simulink library "BatteryPack_lib"  (R2022b)
settings: Solver=VariableStepAuto  StartTime=0.0  StopTime=10.0  RelTol=1e-3
undefined symbols (not defined in the file or in its folder): Battery, ts
libraries: fl_lib x78, nesl_utility x48, simulink x16, batteryecm_lib x14, ee_lib x4
(part 2 of 2)

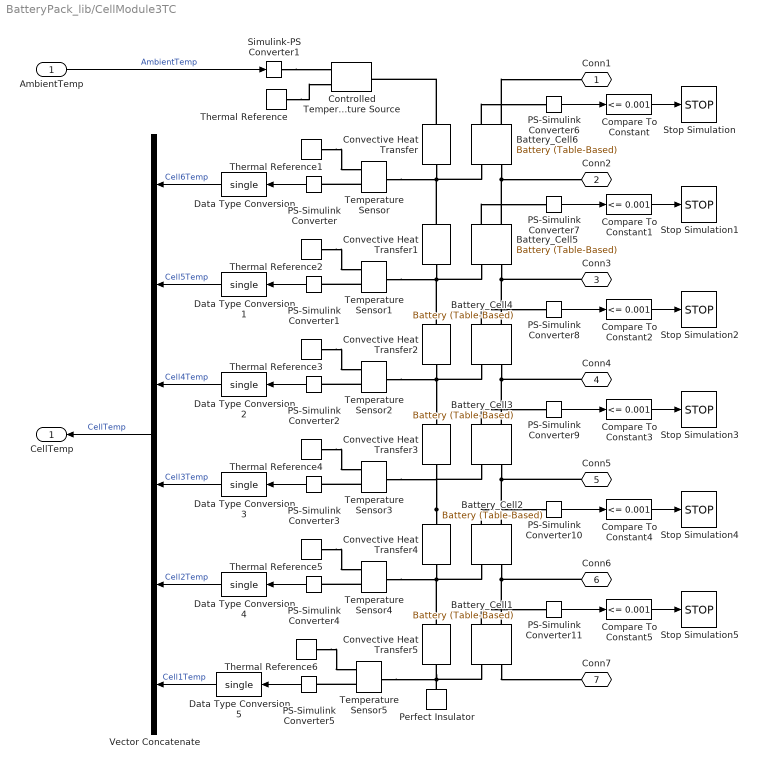
== system BatteryPack_lib/CellModule3TC ==
  AmbientTemp : Inport
  Battery_Cell{1..6} (6 alike) : batteryecm_lib/Battery (Table-Based)  SOC_vec=Battery.SOC_LUT  T_dependence=simscape.enum.tablebattery.temperature_dependence.yes  prm_dir=simscape.enum.tablebattery.prm_dir.noCurrentDirectionality  T_vec=Battery.Temperature_LUT K  V0_mat=Battery.Em_LUT V  V0_vec=[3.1, 3.27, 3.31, 3.5] V  V_range=[0, inf] V  R0_mat=Battery.R0_LUT Ohm  R0_vec=[.015, .017, .012, .013] Ohm  R0_dis_mat=[.0117, .0085, .009; .011, .0085, .009; .0114, .0087, .0092; .0107, .0082, .0088; .0107, .0083, .0091; .0113, .0085, .0089; .0116, .0085, .0089] Ohm  R0_dis_vec=[.0085, .0085, .0087, .0082, .0083, .0085, .0085] Ohm  R0_ch_mat=[.0117, .0085, .009; .011, .0085, .009; .0114, .0087, .0092; .0107, .0082, .0088; .0107, .0083, .0091; .0113, .0085, .0089; .0116, .0085, .0089] Ohm  R0_ch_vec=[.0085, .0085, .0087, .0082, .0083, .0085, .0085] Ohm  AH=Battery.Capacity_LUT hr*A  prm_leak=1  Rleak_vec=[8000, 7000, 6000] Ohm  Rleak=7e3 Ohm  extrapolation_option=simscape.enum.extrapolation.linear  SOC_port=simscape.enum.tablebattery.enable.yes  prm_dyn=4  R1_mat=Battery.R1_LUT Ohm  R1_vec=[.076, .022, .007, .043] Ohm  tau1_mat=Battery.R1_LUT.*Battery.C1_LUT s  tau1_vec=[148, 110, 27, 22] s  R2_mat=Battery.R2_LUT Ohm  R2_vec=[.382, .006, .007, .956] Ohm  tau2_mat=Battery.R2_LUT.*Battery.C2_LUT s  tau2_vec=[44, 24, 14, 13419] s  R3_mat=Battery.R3_LUT Ohm  R3_vec=[.382, .006, .007, .956] Ohm  tau3_mat=Battery.R3_LUT.*Battery.C3_LUT s  tau3_vec=[44, 24, 14, 13419] s  R4_mat=[.014, .382, .407; .028, .006, .007; .014, .007, .006; .333, .956, .912] Ohm  R4_vec=[.382, .006, .007, .956] Ohm  tau4_mat=[1, 44, 5644; 11, 24, 506; 2, 14, 330; 3310, 13419, 30216] s  tau4_vec=[44, 24, 14, 13419] s  R5_mat=[.014, .382, .407; .028, .006, .007; .014, .007, .006; .333, .956, .912] Ohm  R5_vec=[.382, .006, .007, .956] Ohm  tau5_mat=[1, 44, 5644; 11, 24, 506; 2, 14, 330; 3310, 13419, 30216] s  tau5_vec=[44, 24, 14, 13419] s  prm_fade=simscape.enum.tablebattery.prm_fade.equations  N0=100  dV0=0  dR0=0  dAH=0  dRleak=0  dR1=0  dR2=0  dR3=0  dR4=0  dR5=0  N0vec=[100, 200, 300]  Tfadevec=[298.15, 323.15] K  dV0vec=[0, 0, 0]  dR0vec=[0, 0, 0]  dAHvec=[0, 0, 0]  dRleakvec=[0, 0, 0]  dR1vec=[0, 0, 0]  dR2vec=[0, 0, 0]  dR3vec=[0, 0, 0]  dR4vec=[0, 0, 0]  dR5vec=[0, 0, 0]  dV0mat=[0, 0; 0, 0; 0, 0]  dR0mat=[0, 0; 0, 0; 0, 0]  dAHmat=[0, 0; 0, 0; 0, 0]  dRleakmat=[0, 0; 0, 0; 0, 0]  dR1mat=[0, 0; 0, 0; 0, 0]  dR2mat=[0, 0; 0, 0; 0, 0]  dR3mat=[0, 0; 0, 0; 0, 0]  dR4mat=[0, 0; 0, 0; 0, 0]  dR5mat=[0, 0; 0, 0; 0, 0]  prm_age_modeling=simscape.enum.tablebattery.prm_age_modeling.equation  storage_dt_age_vec=[0] d  storage_T_age_vec=[273] K  prm_age_OCV=simscape.enum.tablebattery.prm_age_OCV.OCV  OCV_age=0.9  SOC_age=0.6  prm_age_resistance=simscape.enum.tablebattery.prm_age.disabled  OCV_scaling_age_resistance=2.2134e6  OCV_offset_age_resistance=1.632e6  temp_exp_age_resistance=0.515833569 V  t_exp_age_resistance=0.75  T_age_vec_resistance=[273.15, 298.15, 323.15] K  dt_age_vec_resistance=[90, 180, 270, 360] d  dR0_age_vec=[0, 0, 0]  t_meas_dR0_age=100 d  dR0_age_mat=[0, 0, 0; 0, 0, 0; 0, 0, 0; 0, 0, 0]  prm_age_capacity=simscape.enum.tablebattery.prm_age.disabled  OCV_scaling_age_capacity=1.5097e07  OCV_offset_age_capacity=8.3625e06  temp_exp_age_capacity=0.6011 V  t_exp_age_capacity=0.75  T_age_vec_capacity=[273.15, 298.15, 323.15] K  dt_age_vec_capacity=[90, 180, 270, 360] d  dAH_age_vec=[0, 0, 0]  t_meas_dAH_age=100 d  dAH_age_mat=[0, 0, 0; 0, 0, 0; 0, 0, 0; 0, 0, 0]  thermal_port=simscape.enum.thermaleffects.model  temperature=Battery.TempInit K  thermal_mass=Battery.cell_mass*Battery.cell_Cp_heat J/K  i_specify=off  i_priority=None  i=0 A  i_nominal_specify=off  i_nominal_unit=A  i_nominal_value=1  v_specify=off  v_priority=None  v=0 V  v_nominal_specify=off  v_nominal_unit=V  v_nominal_value=1  stateOfCharge_specify=on  stateOfCharge_priority=High  stateOfCharge=(Battery.Capacity_LUT - Battery.Qe_init)/Battery.Capacity_LUT  stateOfCharge_nominal_specify=off  stateOfCharge_nominal_unit=1  stateOfCharge_nominal_value=1  num_cycles_specify=off  num_cycles_priority=High  num_cycles=0  num_cycles_nominal_specify=off  num_cycles_nominal_unit=1  num_cycles_nominal_value=1  cell_temperature_specify=on  cell_temperature_priority=High  cell_temperature=Battery.TempInit K  cell_temperature_nominal_specify=off  cell_temperature_nominal_unit=K  cell_temperature_nominal_value=1
  Compare To Constant{,1..5} (6 alike) : simulink/Logic and Bit Operations/Compare To Constant  relop=<=  const=0.001  OutDataTypeStr=boolean
  Controlled Temperature Source : fl_lib/Thermal/Thermal Sources/Controlled Temperature Source
  Convective Heat Transfer{,1..5} (6 alike) : fl_lib/Thermal/Thermal Elements/Convective Heat Transfer  thermal_type=foundation.enum.constant_variable.constant  area=Battery.cell_area m^2  heat_tr_coeff=Battery.h_conv W/(m^2 * K)  min_heat_tr_coeff=1e-3 W/(K*m^2)  T_specify=off  T_priority=None  T=0 K  T_nominal_specify=off  T_nominal_unit=K  T_nominal_value=1  Q_specify=off  Q_priority=None  Q=0 W  Q_nominal_specify=off  Q_nominal_unit=W  Q_nominal_value=1
  Data Type Conversion{,1..5} (6 alike) : DataTypeConversion  OutDataTypeStr=single  SaturateOnIntegerOverflow=off  RndMeth=Floor
  PS-Simulink Converter{,1..5} (6 alike) : nesl_utility/PS-Simulink Converter  PhysicalDomain=network_engine_domain  SubClassName=ps_output  LeftPortType=input  RightPortType=output  PseudoPeriodic=off  Frequencies=[]  VectorFormat=1-D array  Unit=K  AffineConversion=off
  PS-Simulink Converter{6..11} (6 alike) : nesl_utility/PS-Simulink Converter  PhysicalDomain=network_engine_domain  SubClassName=ps_output  LeftPortType=input  RightPortType=output  PseudoPeriodic=off  Frequencies=[]  VectorFormat=1-D array  Unit=1  AffineConversion=off
  Perfect Insulator : fl_lib/Thermal/Thermal Elements/Perfect Insulator  T_specify=off  T_priority=None  T=0 K  T_nominal_specify=off  T_nominal_unit=K  T_nominal_value=1
  Simulink-PS Converter1 : nesl_utility/Simulink-PS Converter  PhysicalDomain=network_engine_domain  SubClassName=ps_input  LeftPortType=input  RightPortType=output  PseudoPeriodic=off  Frequencies=[]  NoiseDistribution=none  NoiseParameters=[]  Unit=1  AffineConversion=off  FilteringAndDerivatives=provide  SimscapeFilterOrder=1  InputFilterTimeConstant=0.001  UdotUserProvided=0
  Stop Simulation{,1..5} (6 alike) : Stop
  Temperature Sensor{,1..5} (6 alike) : fl_lib/Thermal/Thermal Sensors/Temperature Sensor
  Thermal Reference{,1..6} (7 alike) : fl_lib/Thermal/Thermal Elements/Thermal Reference
  Vector Concatenate : Concatenate  NumInputs=6
  Conn1 : PMIOPort  Side=Right
  Conn2 : PMIOPort  Port=2  Side=Right
  Conn3 : PMIOPort  Port=3  Side=Right
  Conn4 : PMIOPort  Port=4  Side=Right
  Conn5 : PMIOPort  Port=5  Side=Right
  Conn6 : PMIOPort  Port=6  Side=Right
  Conn7 : PMIOPort  Port=7  Side=Right
  CellTemp : Outport  VectorParamsAs1DForOutWhenUnconnected=off
  wires:
  Compare To Constant3/1 -> Stop Simulation3/1
  Data Type Conversion4/1 -> Vector Concatenate/5  "Cell2Temp"
  Compare To Constant5/1 -> Stop Simulation5/1
  Data Type Conversion5/1 -> Vector Concatenate/6  "Cell1Temp"
  PS-Simulink Converter2/1 -> Data Type Conversion2/1
  Compare To Constant1/1 -> Stop Simulation1/1
  PS-Simulink Converter11/1 -> Compare To Constant5/1
  Data Type Conversion1/1 -> Vector Concatenate/2  "Cell5Temp"
  Compare To Constant4/1 -> Stop Simulation4/1
  Data Type Conversion2/1 -> Vector Concatenate/3  "Cell4Temp"
  Data Type Conversion3/1 -> Vector Concatenate/4  "Cell3Temp"
  PS-Simulink Converter8/1 -> Compare To Constant2/1
  PS-Simulink Converter3/1 -> Data Type Conversion3/1
  PS-Simulink Converter1/1 -> Data Type Conversion1/1
  PS-Simulink Converter9/1 -> Compare To Constant3/1
  PS-Simulink Converter4/1 -> Data Type Conversion4/1
  PS-Simulink Converter10/1 -> Compare To Constant4/1
  PS-Simulink Converter7/1 -> Compare To Constant1/1
  PS-Simulink Converter5/1 -> Data Type Conversion5/1
  Compare To Constant/1 -> Stop Simulation/1
  PS-Simulink Converter/1 -> Data Type Conversion/1
  Data Type Conversion/1 -> Vector Concatenate/1  "Cell6Temp"
  Compare To Constant2/1 -> Stop Simulation2/1
  AmbientTemp/1 -> Simulink-PS Converter1/1  "AmbientTemp"
  Vector Concatenate/1 -> CellTemp/1  "CellTemp"
  PS-Simulink Converter6/1 -> Compare To Constant/1
  connections:
  Battery_Cell3/RConn1 -- Conn5/RConn1 -- Battery_Cell2/LConn1
  Temperature Sensor2/RConn2 -- PS-Simulink Converter2/LConn1
  Battery_Cell1/LConn2 -- PS-Simulink Converter11/LConn1
  Temperature Sensor1/RConn2 -- PS-Simulink Converter1/LConn1
  Battery_Cell2/RConn1 -- Conn6/RConn1 -- Battery_Cell1/LConn1
  Battery_Cell4/RConn1 -- Conn4/RConn1 -- Battery_Cell3/LConn1
  Convective Heat Transfer/LConn1 -- Controlled Temperature Source/LConn1
  Thermal Reference1/LConn1 -- Temperature Sensor/RConn1
  Convective Heat Transfer1/LConn1 -- Temperature Sensor/LConn1 -- Convective Heat Transfer/RConn1 -- Battery_Cell6/RConn2
  Convective Heat Transfer5/LConn1 -- Temperature Sensor4/LConn1 -- Convective Heat Transfer4/RConn1 -- Battery_Cell2/RConn2
  Battery_Cell6/RConn1 -- Conn2/RConn1 -- Battery_Cell5/LConn1
  Perfect Insulator/LConn1 -- Temperature Sensor5/LConn1 -- Convective Heat Transfer5/RConn1 -- Battery_Cell1/RConn2
  Thermal Reference3/LConn1 -- Temperature Sensor2/RConn1
  Temperature Sensor/RConn2 -- PS-Simulink Converter/LConn1
  Convective Heat Transfer4/LConn1 -- Temperature Sensor3/LConn1 -- Convective Heat Transfer3/RConn1 -- Battery_Cell3/RConn2
  Battery_Cell1/RConn1 -- Conn7/RConn1
  Battery_Cell6/LConn1 -- Conn1/RConn1
  Battery_Cell6/LConn2 -- PS-Simulink Converter6/LConn1
  Thermal Reference4/LConn1 -- Temperature Sensor3/RConn1
  Temperature Sensor3/RConn2 -- PS-Simulink Converter3/LConn1
  Thermal Reference5/LConn1 -- Temperature Sensor4/RConn1
  Thermal Reference/LConn1 -- Controlled Temperature Source/RConn2
  Temperature Sensor4/RConn2 -- PS-Simulink Converter4/LConn1
  Battery_Cell4/RConn2 -- Temperature Sensor2/LConn1 -- Convective Heat Transfer2/RConn1 -- Convective Heat Transfer3/LConn1
  Temperature Sensor5/RConn2 -- PS-Simulink Converter5/LConn1
  Thermal Reference6/LConn1 -- Temperature Sensor5/RConn1
  Battery_Cell5/RConn1 -- Conn3/RConn1 -- Battery_Cell4/LConn1
  Battery_Cell5/LConn2 -- PS-Simulink Converter7/LConn1
  Convective Heat Transfer2/LConn1 -- Temperature Sensor1/LConn1 -- Convective Heat Transfer1/RConn1 -- Battery_Cell5/RConn2
  Battery_Cell3/LConn2 -- PS-Simulink Converter9/LConn1
  Battery_Cell4/LConn2 -- PS-Simulink Converter8/LConn1
  Battery_Cell2/LConn2 -- PS-Simulink Converter10/LConn1
  Thermal Reference2/LConn1 -- Temperature Sensor1/RConn1
  Simulink-PS Converter1/RConn1 -- Controlled Temperature Source/RConn1

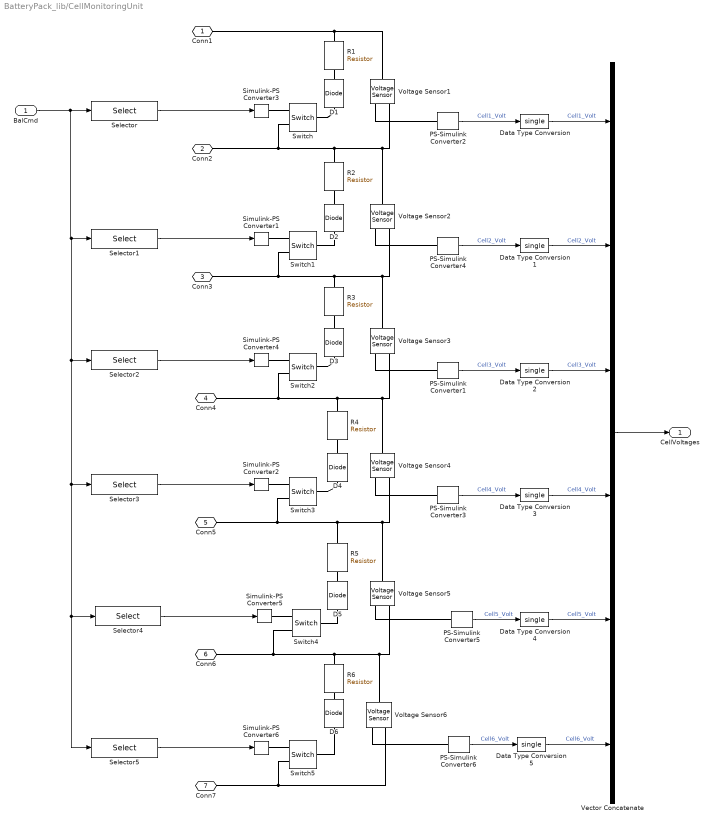
== system BatteryPack_lib/CellMonitoringUnit ==
  BalCmd : Inport
  D{1..4} (4 alike) : fl_lib/Electrical/Electrical Elements/Diode  Vf=0.6 V  Ron=0.3 Ohm  Goff=1e-8 1/Ohm  i_specify=off  i_priority=High  i=0 A  i_nominal_specify=off  i_nominal_unit=A  i_nominal_value=1  v_specify=off  v_priority=None  v=0 V  v_nominal_specify=off  v_nominal_unit=V  v_nominal_value=1
      settings: LogSimulationData=on
  D5 : fl_lib/Electrical/Electrical Elements/Diode  Vf=0.6 V  Ron=0.3 Ohm  Goff=1e-8 1/Ohm  i_specify=off  i_priority=None  i=0 A  i_nominal_specify=off  i_nominal_unit=A  i_nominal_value=1  v_specify=off  v_priority=None  v=0 V  v_nominal_specify=off  v_nominal_unit=V  v_nominal_value=1
      settings: LogSimulationData=on
  D6 : fl_lib/Electrical/Electrical Elements/Diode  Vf=0.6 V  Ron=0.3 Ohm  Goff=1e-8 1/Ohm  i_specify=off  i_priority=None  i=0 A  i_nominal_specify=off  i_nominal_unit=A  i_nominal_value=1  v_specify=off  v_priority=None  v=0 V  v_nominal_specify=off  v_nominal_unit=V  v_nominal_value=1
      settings: LogSimulationData=on
  Data Type Conversion{,1..5} (6 alike) : DataTypeConversion  OutDataTypeStr=single  SaturateOnIntegerOverflow=off  RndMeth=Floor
  PS-Simulink Converter{1..6} (6 alike) : nesl_utility/PS-Simulink Converter  PhysicalDomain=network_engine_domain  SubClassName=ps_output  LeftPortType=input  RightPortType=output  PseudoPeriodic=off  Frequencies=[]  VectorFormat=1-D array  Unit=V  AffineConversion=off
  R{1..6} (6 alike) : fl_lib/Electrical/Electrical Elements/Resistor  R=Battery.R_bleed Ohm  i_specify=off  i_priority=None  i=0 A  i_nominal_specify=off  i_nominal_unit=A  i_nominal_value=1  v_specify=off  v_priority=None  v=0 V  v_nominal_specify=off  v_nominal_unit=V  v_nominal_value=1
      R1 settings: LogSimulationData=on
  Selector : Selector  IndexOptions=Index vector (dialog)  Indices=1  OutputSizes=1
  Selector1 : Selector  IndexOptions=Index vector (dialog)  Indices=2  OutputSizes=1
  Selector2 : Selector  IndexOptions=Index vector (dialog)  Indices=3  OutputSizes=1
  Selector3 : Selector  IndexOptions=Index vector (dialog)  Indices=4  OutputSizes=1
  Selector4 : Selector  IndexOptions=Index vector (dialog)  Indices=5  OutputSizes=1
  Selector5 : Selector  IndexOptions=Index vector (dialog)  Indices=6  OutputSizes=1
  Simulink-PS Converter{1..6} (6 alike) : nesl_utility/Simulink-PS Converter  PhysicalDomain=network_engine_domain  SubClassName=ps_input  LeftPortType=input  RightPortType=output  PseudoPeriodic=off  Frequencies=[]  NoiseDistribution=none  NoiseParameters=[]  Unit=1  AffineConversion=off  FilteringAndDerivatives=zero  SimscapeFilterOrder=1  InputFilterTimeConstant=0.001  UdotUserProvided=1
  Switch{,1..5} (6 alike) : fl_lib/Electrical/Electrical Elements/Switch  R_closed=0.01 Ohm  G_open=1e-8 1/Ohm  Threshold=0  i_specify=off  i_priority=None  i=0 A  i_nominal_specify=off  i_nominal_unit=A  i_nominal_value=1  v_specify=off  v_priority=None  v=0 V  v_nominal_specify=off  v_nominal_unit=V  v_nominal_value=1
  Vector Concatenate : Concatenate  NumInputs=6
  Voltage Sensor{1..6} (6 alike) : fl_lib/Electrical/Electrical Sensors/Voltage Sensor
  Conn1 : PMIOPort  Side=Left
  Conn2 : PMIOPort  Port=2  Side=Left
  Conn3 : PMIOPort  Port=3  Side=Left
  Conn4 : PMIOPort  Port=4  Side=Left
  Conn5 : PMIOPort  Port=5  Side=Left
  Conn6 : PMIOPort  Port=6  Side=Left
  Conn7 : PMIOPort  Port=7  Side=Left
  CellVoltages : Outport  VectorParamsAs1DForOutWhenUnconnected=off
  wires:
  Vector Concatenate/1 -> CellVoltages/1
  Selector2/1 -> Simulink-PS Converter4/1
  Selector1/1 -> Simulink-PS Converter1/1
  BalCmd/1 -> Selector5/1, Selector4/1, Selector3/1, Selector2/1, Selector1/1, Selector/1
  PS-Simulink Converter2/1 -> Data Type Conversion/1  "Cell1_Volt"
  PS-Simulink Converter1/1 -> Data Type Conversion2/1  "Cell3_Volt"
  PS-Simulink Converter4/1 -> Data Type Conversion1/1  "Cell2_Volt"
  Selector/1 -> Simulink-PS Converter3/1
  Selector3/1 -> Simulink-PS Converter2/1
  Selector4/1 -> Simulink-PS Converter5/1
  Selector5/1 -> Simulink-PS Converter6/1
  PS-Simulink Converter3/1 -> Data Type Conversion3/1  "Cell4_Volt"
  PS-Simulink Converter5/1 -> Data Type Conversion4/1  "Cell5_Volt"
  PS-Simulink Converter6/1 -> Data Type Conversion5/1  "Cell6_Volt"
  Data Type Conversion/1 -> Vector Concatenate/1  "Cell1_Volt"
  Data Type Conversion1/1 -> Vector Concatenate/2  "Cell2_Volt"
  Data Type Conversion2/1 -> Vector Concatenate/3  "Cell3_Volt"
  Data Type Conversion3/1 -> Vector Concatenate/4  "Cell4_Volt"
  Data Type Conversion4/1 -> Vector Concatenate/5  "Cell5_Volt"
  Data Type Conversion5/1 -> Vector Concatenate/6  "Cell6_Volt"
  connections:
  Voltage Sensor3/RConn2 -- Voltage Sensor4/LConn1 -- R4/LConn1 -- Conn4/RConn1 -- Switch2/RConn2
  Voltage Sensor3/RConn1 -- PS-Simulink Converter1/LConn1
  Simulink-PS Converter4/RConn1 -- Switch2/RConn1
  Simulink-PS Converter1/RConn1 -- Switch1/RConn1
  Simulink-PS Converter3/RConn1 -- Switch/RConn1
  Switch1/LConn1 -- D2/RConn1
  Voltage Sensor2/RConn1 -- PS-Simulink Converter4/LConn1
  PS-Simulink Converter2/LConn1 -- Voltage Sensor1/RConn1
  Conn1/RConn1 -- Voltage Sensor1/LConn1 -- R1/LConn1
  Switch2/LConn1 -- D3/RConn1
  Switch/LConn1 -- D1/RConn1
  R2/RConn1 -- D2/LConn1
  R1/RConn1 -- D1/LConn1
  Conn2/RConn1 -- Voltage Sensor1/RConn2 -- Voltage Sensor2/LConn1 -- R2/LConn1 -- Switch/RConn2
  Voltage Sensor2/RConn2 -- Voltage Sensor3/LConn1 -- Conn3/RConn1 -- Switch1/RConn2 -- R3/LConn1
  R3/RConn1 -- D3/LConn1
  R5/LConn1 -- Conn5/RConn1 -- Switch3/RConn2 -- Voltage Sensor5/LConn1 -- Voltage Sensor4/RConn2
  R4/RConn1 -- D4/LConn1
  Switch3/LConn1 -- D4/RConn1
  Simulink-PS Converter2/RConn1 -- Switch3/RConn1
  Conn6/RConn1 -- Switch4/RConn2 -- Voltage Sensor5/RConn2 -- Voltage Sensor6/LConn1 -- R6/LConn1
  Simulink-PS Converter5/RConn1 -- Switch4/RConn1
  R5/RConn1 -- D5/LConn1
  Switch4/LConn1 -- D5/RConn1
  Voltage Sensor6/RConn2 -- Conn7/RConn1 -- Switch5/RConn2
  Switch5/LConn1 -- D6/RConn1
  Simulink-PS Converter6/RConn1 -- Switch5/RConn1
  R6/RConn1 -- D6/LConn1
  Voltage Sensor4/RConn1 -- PS-Simulink Converter3/LConn1
  Voltage Sensor5/RConn1 -- PS-Simulink Converter5/LConn1
  Voltage Sensor6/RConn1 -- PS-Simulink Converter6/LConn1

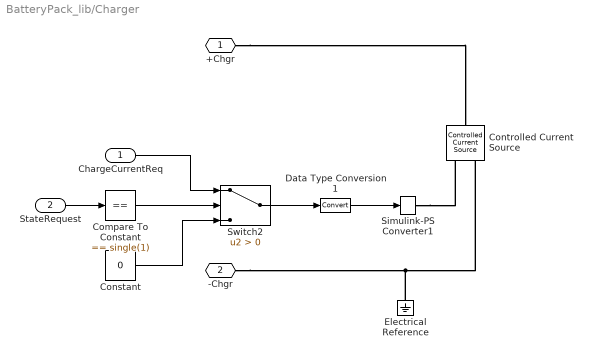
== system BatteryPack_lib/Charger ==
  ChargeCurrentReq : Inport
  StateRequest : Inport  Port=2
  Compare To Constant : simulink/Logic and Bit Operations/Compare To Constant  relop===  const=single(1)  OutDataTypeStr=boolean
  Constant : Constant  Value=0  SampleTime=ts
  Controlled Current Source : fl_lib/Electrical/Electrical Sources/Controlled Current Source
      settings: LogSimulationData=on
  Data Type Conversion1 : DataTypeConversion  SaturateOnIntegerOverflow=off  RndMeth=Floor
  Electrical Reference : fl_lib/Electrical/Electrical Elements/Electrical Reference
  Simulink-PS Converter1 : nesl_utility/Simulink-PS Converter  PhysicalDomain=network_engine_domain  SubClassName=ps_input  LeftPortType=input  RightPortType=output  PseudoPeriodic=off  Frequencies=[]  NoiseDistribution=none  NoiseParameters=[]  Unit=A  AffineConversion=off  FilteringAndDerivatives=zero  SimscapeFilterOrder=1  InputFilterTimeConstant=0.1  UdotUserProvided=1
  Switch2 : Switch  Criteria=u2 > Threshold  SaturateOnIntegerOverflow=off  InputSameDT=off
  +Chgr : PMIOPort  Side=Left
  -Chgr : PMIOPort  Port=2  Side=Left
  wires:
  Compare To Constant/1 -> Switch2/2
  Switch2/1 -> Data Type Conversion1/1
  Constant/1 -> Switch2/3
  StateRequest/1 -> Compare To Constant/1
  Data Type Conversion1/1 -> Simulink-PS Converter1/1
  ChargeCurrentReq/1 -> Switch2/1
  connections:
  +Chgr/RConn1 -- Controlled Current Source/LConn1
  Controlled Current Source/RConn2 -- -Chgr/RConn1 -- Electrical Reference/LConn1
  Simulink-PS Converter1/RConn1 -- Controlled Current Source/RConn1

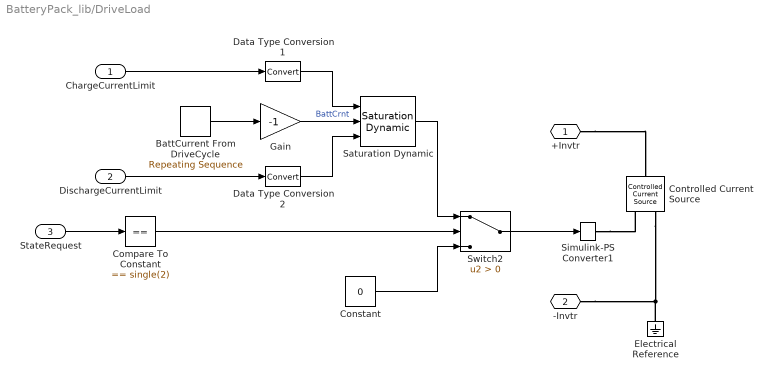
== system BatteryPack_lib/DriveLoad ==
  ChargeCurrentLimit : Inport
  DischargeCurrentLimit : Inport  Port=2
  StateRequest : Inport  Port=3
  BattCurrent From DriveCycle : simulink/Sources/Repeating Sequence  rep_seq_t=BattCrnt.Time  rep_seq_y=BattCrnt.Data
  Compare To Constant : simulink/Logic and Bit Operations/Compare To Constant  relop===  const=single(2)  OutDataTypeStr=boolean
  Constant : Constant  Value=0  SampleTime=ts
  Controlled Current Source : fl_lib/Electrical/Electrical Sources/Controlled Current Source
      settings: LogSimulationData=on
  Data Type Conversion1 : DataTypeConversion  SaturateOnIntegerOverflow=off  RndMeth=Floor
  Data Type Conversion2 : DataTypeConversion  SaturateOnIntegerOverflow=off  RndMeth=Floor
  Electrical Reference : fl_lib/Electrical/Electrical Elements/Electrical Reference
  Gain : Gain  Gain=-1
  Saturation Dynamic : simulink/Discontinuities/Saturation Dynamic  OutMin=[]  OutMax=[]  OutDataTypeStr=Inherit: Same as second input  OutDataType=fixdt(1, 16)  OutScaling=2^-10  DoSatur=off
  Simulink-PS Converter1 : nesl_utility/Simulink-PS Converter  PhysicalDomain=network_engine_domain  SubClassName=ps_input  LeftPortType=input  RightPortType=output  PseudoPeriodic=off  Frequencies=[]  NoiseDistribution=none  NoiseParameters=[]  Unit=A  AffineConversion=off  FilteringAndDerivatives=zero  SimscapeFilterOrder=1  InputFilterTimeConstant=0.1  UdotUserProvided=1
  Switch2 : Switch  Criteria=u2 > Threshold  SaturateOnIntegerOverflow=off  InputSameDT=off
  +Invtr : PMIOPort  Side=Left
  -Invtr : PMIOPort  Port=2  Side=Left
  wires:
  BattCurrent From DriveCycle/1 -> Gain/1
  Gain/1 -> Saturation Dynamic/2  "BattCrnt"
  Compare To Constant/1 -> Switch2/2
  StateRequest/1 -> Compare To Constant/1
  Switch2/1 -> Simulink-PS Converter1/1
  Constant/1 -> Switch2/3
  Data Type Conversion2/1 -> Saturation Dynamic/3
  Data Type Conversion1/1 -> Saturation Dynamic/1
  ChargeCurrentLimit/1 -> Data Type Conversion1/1
  DischargeCurrentLimit/1 -> Data Type Conversion2/1
  Saturation Dynamic/1 -> Switch2/1
  connections:
  Simulink-PS Converter1/RConn1 -- Controlled Current Source/RConn1
  -Invtr/RConn1 -- Electrical Reference/LConn1 -- Controlled Current Source/RConn2
  +Invtr/RConn1 -- Controlled Current Source/LConn1

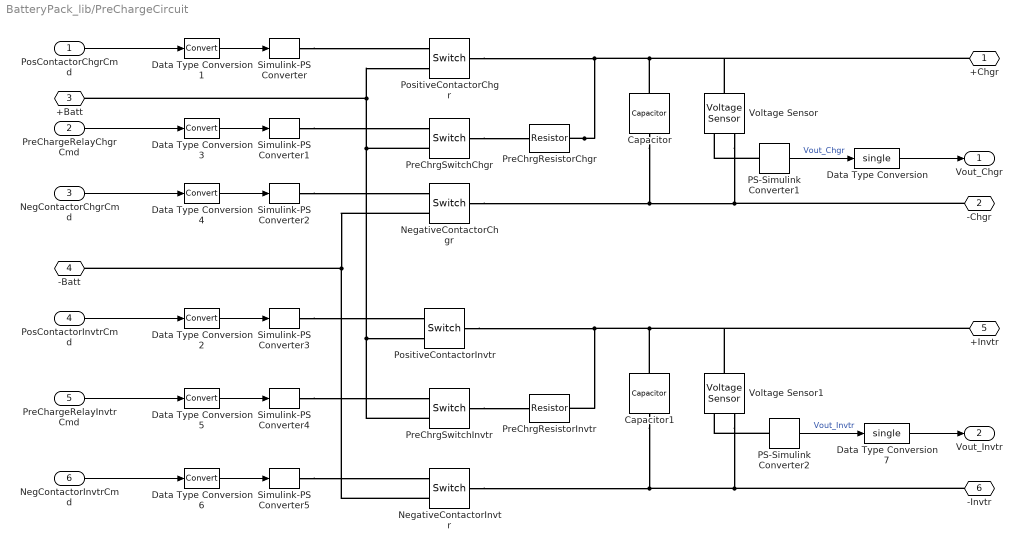
== system BatteryPack_lib/PreChargeCircuit ==
  PosContactorChgrCmd : Inport
  PreChargeRelayChgrCmd : Inport  Port=2
  NegContactorChgrCmd : Inport  Port=3
  PosContactorInvtrCmd : Inport  Port=4
  PreChargeRelayInvtrCmd : Inport  Port=5
  NegContactorInvtrCmd : Inport  Port=6
  Capacitor : ee_lib/Passive/Capacitor  cap_option=0  c=10000 uF  Cvec=[1e-05, 1e-06] F  Vvec=[0, 10] V  CV_table_symmetry=1  f_vec=[1, 10] kHz  DFext_vec=[.8, 1.2]  enable_C_tol=0  C_tol=5  tol_distribution=1  nSigma=4  r=1e-9 Ohm  g=0 1/Ohm  averaging_period=0 s  enable_operating_limits=0  operating_limit_action=2  max_working_voltage_range=[-25, 25] V  power_rating=1 W  enable_faults=0  fault_action=1  Cscale_faulted=100  R_faulted=1e-3 Ohm  G_faulted=0 1/Ohm  tau_fault=1e-3 s  enable_temporal_fault=0  t_fault=1 s  enable_behavioral_fault=0  max_permissible_voltage_range=[-100, 100] V  t_fail_on_voltage=1 s  i_specify=off  i_priority=None  i=0 A  i_nominal_specify=off  i_nominal_unit=A  i_nominal_value=1  v_specify=off  v_priority=None  v=0 V  v_nominal_specify=off  v_nominal_unit=V  v_nominal_value=1  vc_specify=off  vc_priority=High  vc=0 V  vc_nominal_specify=off  vc_nominal_unit=V  vc_nominal_value=1
  Capacitor1 : ee_lib/Passive/Capacitor  cap_option=0  c=10000 uF  Cvec=[1e-05, 1e-06] F  Vvec=[0, 10] V  CV_table_symmetry=1  f_vec=[1, 10] kHz  DFext_vec=[.8, 1.2]  enable_C_tol=0  C_tol=5  tol_distribution=1  nSigma=4  r=1e-9 Ohm  g=0 1/Ohm  averaging_period=0 s  enable_operating_limits=0  operating_limit_action=2  max_working_voltage_range=[-25, 25] V  power_rating=1 W  enable_faults=0  fault_action=1  Cscale_faulted=100  R_faulted=1e-3 Ohm  G_faulted=0 1/Ohm  tau_fault=1e-3 s  enable_temporal_fault=0  t_fault=1 s  enable_behavioral_fault=0  max_permissible_voltage_range=[-100, 100] V  t_fail_on_voltage=1 s  i_specify=off  i_priority=None  i=0 A  i_nominal_specify=off  i_nominal_unit=A  i_nominal_value=1  v_specify=off  v_priority=None  v=0 V  v_nominal_specify=off  v_nominal_unit=V  v_nominal_value=1  vc_specify=off  vc_priority=High  vc=0 V  vc_nominal_specify=off  vc_nominal_unit=V  vc_nominal_value=1
  Data Type Conversion : DataTypeConversion  OutDataTypeStr=single  SaturateOnIntegerOverflow=off  RndMeth=Floor
  Data Type Conversion{1..6} (6 alike) : DataTypeConversion  SaturateOnIntegerOverflow=off  RndMeth=Floor
  Data Type Conversion7 : DataTypeConversion  OutDataTypeStr=single  SaturateOnIntegerOverflow=off  RndMeth=Floor
  NegativeContactorChgr : fl_lib/Electrical/Electrical Elements/Switch  R_closed=0.01 Ohm  G_open=1e-8 1/Ohm  Threshold=0  i_specify=off  i_priority=None  i=0 A  i_nominal_specify=off  i_nominal_unit=A  i_nominal_value=1  v_specify=off  v_priority=None  v=0 V  v_nominal_specify=off  v_nominal_unit=V  v_nominal_value=1
  NegativeContactorInvtr : fl_lib/Electrical/Electrical Elements/Switch  R_closed=0.01 Ohm  G_open=1e-8 1/Ohm  Threshold=0  i_specify=off  i_priority=None  i=0 A  i_nominal_specify=off  i_nominal_unit=A  i_nominal_value=1  v_specify=off  v_priority=None  v=0 V  v_nominal_specify=off  v_nominal_unit=V  v_nominal_value=1
  PS-Simulink Converter1 : nesl_utility/PS-Simulink Converter  PhysicalDomain=network_engine_domain  SubClassName=ps_output  LeftPortType=input  RightPortType=output  PseudoPeriodic=off  Frequencies=[]  VectorFormat=1-D array  Unit=V  AffineConversion=off
  PS-Simulink Converter2 : nesl_utility/PS-Simulink Converter  PhysicalDomain=network_engine_domain  SubClassName=ps_output  LeftPortType=input  RightPortType=output  PseudoPeriodic=off  Frequencies=[]  VectorFormat=1-D array  Unit=V  AffineConversion=off
  PositiveContactorChgr : fl_lib/Electrical/Electrical Elements/Switch  R_closed=0.0001 Ohm  G_open=1e-8 1/Ohm  Threshold=0.9  i_specify=off  i_priority=None  i=0 A  i_nominal_specify=off  i_nominal_unit=A  i_nominal_value=1  v_specify=off  v_priority=None  v=0 V  v_nominal_specify=off  v_nominal_unit=V  v_nominal_value=1
  PositiveContactorInvtr : fl_lib/Electrical/Electrical Elements/Switch  R_closed=0.0001 Ohm  G_open=1e-8 1/Ohm  Threshold=0.9  i_specify=off  i_priority=None  i=0 A  i_nominal_specify=off  i_nominal_unit=A  i_nominal_value=1  v_specify=off  v_priority=None  v=0 V  v_nominal_specify=off  v_nominal_unit=V  v_nominal_value=1
  PreChrgResistorChgr : ee_lib/Passive/Resistor  R=20 Ohm  enable_R_tol=0  R_tol=5  tol_distribution=1  nSigma=4  enable_operating_limits=0  operating_limit_action=2  max_working_voltage=100 V  power_rating=1 W  enable_faults=0  fault_action=1  R_faulted=inf Ohm  enable_temporal_fault=0  t_fault=1 s  enable_behavioral_fault=0  max_permissible_current=1 A  t_fail_on_current=1 s  noise_mode=0  sample_time=1e-3 s  repeatability=1  auto_seed=3933054132  user_seed=0  Tdevice=25 degC  power_derating_T1=70 degC  power_derating_T2=155 degC  operating_temperature_range_vec=[-50, 150] degC  alpha=3.93e-3 1/K  Tmeas=25 degC  thermal_mass=100 J/K  temperature_specify=off  temperature_priority=High  temperature=298.15 K  temperature_nominal_specify=off  temperature_nominal_unit=K  temperature_nominal_value=1
  PreChrgResistorInvtr : ee_lib/Passive/Resistor  R=20 Ohm  enable_R_tol=0  R_tol=5  tol_distribution=1  nSigma=4  enable_operating_limits=0  operating_limit_action=2  max_working_voltage=100 V  power_rating=1 W  enable_faults=0  fault_action=1  R_faulted=inf Ohm  enable_temporal_fault=0  t_fault=1 s  enable_behavioral_fault=0  max_permissible_current=1 A  t_fail_on_current=1 s  noise_mode=0  sample_time=1e-3 s  repeatability=1  auto_seed=3402504572  user_seed=0  Tdevice=25 degC  power_derating_T1=70 degC  power_derating_T2=155 degC  operating_temperature_range_vec=[-50, 150] degC  alpha=3.93e-3 1/K  Tmeas=25 degC  thermal_mass=100 J/K  temperature_specify=off  temperature_priority=High  temperature=298.15 K  temperature_nominal_specify=off  temperature_nominal_unit=K  temperature_nominal_value=1
  PreChrgSwitchChgr : fl_lib/Electrical/Electrical Elements/Switch  R_closed=0.0001 Ohm  G_open=1e-8 1/Ohm  Threshold=0.9  i_specify=off  i_priority=None  i=0 A  i_nominal_specify=off  i_nominal_unit=A  i_nominal_value=1  v_specify=off  v_priority=None  v=0 V  v_nominal_specify=off  v_nominal_unit=V  v_nominal_value=1
  PreChrgSwitchInvtr : fl_lib/Electrical/Electrical Elements/Switch  R_closed=0.0001 Ohm  G_open=1e-8 1/Ohm  Threshold=0.9  i_specify=off  i_priority=None  i=0 A  i_nominal_specify=off  i_nominal_unit=A  i_nominal_value=1  v_specify=off  v_priority=None  v=0 V  v_nominal_specify=off  v_nominal_unit=V  v_nominal_value=1
  Simulink-PS Converter{,1..5} (6 alike) : nesl_utility/Simulink-PS Converter  PhysicalDomain=network_engine_domain  SubClassName=ps_input  LeftPortType=input  RightPortType=output  PseudoPeriodic=off  Frequencies=[]  NoiseDistribution=none  NoiseParameters=[]  Unit=1  AffineConversion=off  FilteringAndDerivatives=provide  SimscapeFilterOrder=1  InputFilterTimeConstant=0.001  UdotUserProvided=0
  Voltage Sensor : fl_lib/Electrical/Electrical Sensors/Voltage Sensor
  Voltage Sensor1 : fl_lib/Electrical/Electrical Sensors/Voltage Sensor
  +Chgr : PMIOPort  Side=Right
  -Chgr : PMIOPort  Port=2  Side=Right
  +Batt : PMIOPort  Port=3  Side=Left
  -Batt : PMIOPort  Port=4  Side=Left
  +Invtr : PMIOPort  Port=5  Side=Right
  -Invtr : PMIOPort  Port=6  Side=Right
  Vout_Chgr : Outport  VectorParamsAs1DForOutWhenUnconnected=off
  Vout_Invtr : Outport  Port=2  VectorParamsAs1DForOutWhenUnconnected=off
  wires:
  Data Type Conversion7/1 -> Vout_Invtr/1
  Data Type Conversion/1 -> Vout_Chgr/1
  PosContactorInvtrCmd/1 -> Data Type Conversion2/1
  PreChargeRelayInvtrCmd/1 -> Data Type Conversion5/1
  NegContactorInvtrCmd/1 -> Data Type Conversion6/1
  Data Type Conversion6/1 -> Simulink-PS Converter5/1
  Data Type Conversion5/1 -> Simulink-PS Converter4/1
  Data Type Conversion2/1 -> Simulink-PS Converter3/1
  PS-Simulink Converter2/1 -> Data Type Conversion7/1  "Vout_Invtr"
  Data Type Conversion1/1 -> Simulink-PS Converter/1
  NegContactorChgrCmd/1 -> Data Type Conversion4/1
  PS-Simulink Converter1/1 -> Data Type Conversion/1  "Vout_Chgr"
  Data Type Conversion3/1 -> Simulink-PS Converter1/1
  Data Type Conversion4/1 -> Simulink-PS Converter2/1
  PosContactorChgrCmd/1 -> Data Type Conversion1/1
  PreChargeRelayChgrCmd/1 -> Data Type Conversion3/1
  connections:
  PS-Simulink Converter2/LConn1 -- Voltage Sensor1/RConn1
  Simulink-PS Converter5/RConn1 -- NegativeContactorInvtr/RConn1
  Simulink-PS Converter3/RConn1 -- PositiveContactorInvtr/RConn1
  PreChrgSwitchInvtr/LConn1 -- PreChrgResistorInvtr/LConn1
  Simulink-PS Converter4/RConn1 -- PreChrgSwitchInvtr/RConn1
  Voltage Sensor1/RConn2 -- NegativeContactorInvtr/LConn1 -- Capacitor1/RConn1 -- -Invtr/RConn1
  PositiveContactorInvtr/LConn1 -- PreChrgResistorInvtr/RConn1 -- +Invtr/RConn1 -- Voltage Sensor1/LConn1 -- Capacitor1/LConn1
  Simulink-PS Converter2/RConn1 -- NegativeContactorChgr/RConn1
  PreChrgSwitchChgr/LConn1 -- PreChrgResistorChgr/LConn1
  Simulink-PS Converter/RConn1 -- PositiveContactorChgr/RConn1
  Simulink-PS Converter1/RConn1 -- PreChrgSwitchChgr/RConn1
  PS-Simulink Converter1/LConn1 -- Voltage Sensor/RConn1
  NegativeContactorInvtr/RConn2 -- -Batt/RConn1 -- NegativeContactorChgr/RConn2
  PreChrgSwitchInvtr/RConn2 -- PreChrgSwitchChgr/RConn2 -- +Batt/RConn1 -- PositiveContactorChgr/RConn2 -- PositiveContactorInvtr/RConn2
  Capacitor/RConn1 -- -Chgr/RConn1 -- Voltage Sensor/RConn2 -- NegativeContactorChgr/LConn1
  PreChrgResistorChgr/RConn1 -- PositiveContactorChgr/LConn1 -- Voltage Sensor/LConn1 -- +Chgr/RConn1 -- Capacitor/LConn1
